simulink model "IP02"  (R2021a)
settings: Solver=VariableStepAuto  StartTime=0.0  StopTime=10.0  RelTol=1e-3
values from neighbouring files (symbols this model uses):
  a = rmp*ng*kg*nm*kt    (= 0.000180693695)    [IP02_DEFINITIVO.m]
  b = Rm*M*rmp^2+Rm*ng*kg^2*jm    (= 7.37147424e-05)    [IP02_DEFINITIVO.m]
  c = ng*kg^2*nm*kt*km+B_eq*Rm*rmp^2    (= 0.00137585476249)    [IP02_DEFINITIVO.m]
  dc = [1 502.2629]    [IP02_DEFINITIVO.m]
  k = K_necesari    [IP02_DEFINITIVO.m]
  nc = [6.2783 80]    [IP02_DEFINITIVO.m]
settings Model: Creator=Equipo  LastModifiedBy=Equipo

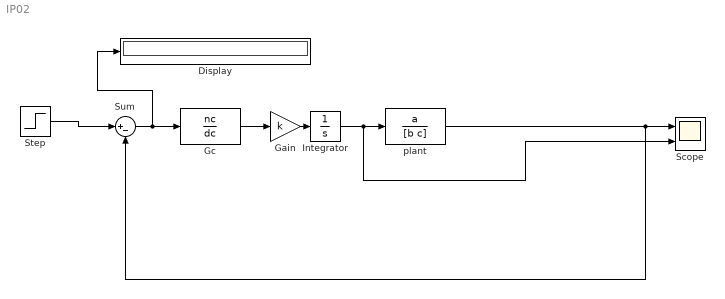
== system IP02 ==
  Display : Display
  Gain : Gain  Gain=k
  Gc : TransferFcn  Numerator=nc  Denominator=dc
  Integrator : Integrator
  Scope : Scope  NumInputPorts=2
  Step : Step  SampleTime=0
  Sum : Sum  Inputs=|+-
  plant : TransferFcn  Numerator=a  Denominator=[b c]
  wires:
  Step/1 -> Sum/1
  Sum/1 -> Gc/1, Display/1
  Gc/1 -> Gain/1
  Gain/1 -> Integrator/1
  plant/1 -> Scope/1, Sum/2
  Integrator/1 -> plant/1, Scope/2
